simulink model "APP"  (R2024a)
settings: Solver=FixedStepAuto  StartTime=0.0  StopTime=10.0  RelTol=1e-3
settings Model: Creator=Bsmala  LastModifiedBy=Bsmala
settings DataIOCC: LoadExternalInput=on

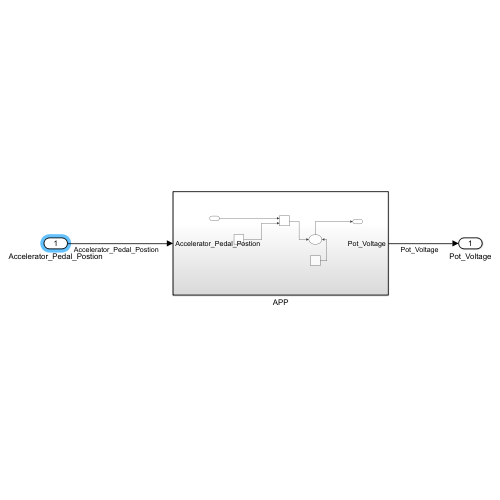
[thumbnail: Simulink's stored preview of the top-level diagram]
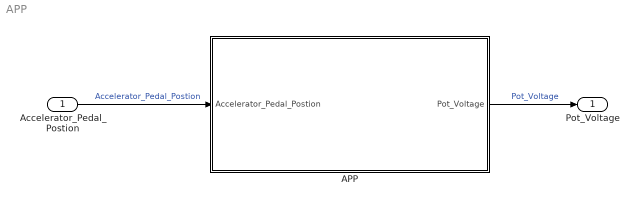
== system APP ==
  Accelerator_Pedal_Postion : Inport
  APP : Subsystem
  Pot_Voltage : Outport
  wires:
  Accelerator_Pedal_Postion/1 -> APP/1(Accelerator_Pedal_Postion)  "Accelerator_Pedal_Postion"
  APP/1(Pot_Voltage) -> Pot_Voltage/1  "Pot_Voltage"

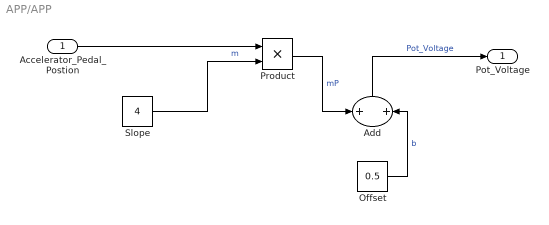
== system APP/APP ==
  Accelerator_Pedal_Postion : Inport
  Add : Sum
  Offset : Constant  Value=0.5
  Product : Product
  Slope : Constant  Value=4
  Pot_Voltage : Outport
  wires:
  Slope/1 -> Product/2  "m"
  Offset/1 -> Add/2  "b"
  Product/1 -> Add/1  "mP"
  Add/1 -> Pot_Voltage/1  "Pot_Voltage"
  Accelerator_Pedal_Postion/1 -> Product/1
